simulink model "task_4_sim"  (R2023a)
settings: Solver=VariableStepAuto  StartTime=0.0  StopTime=10.0  RelTol=1e-3
undefined symbols (not defined in the file): A, B, Cz, Dz, G, K1, K2, w0
settings Model: Creator=user  LastModifiedBy=user

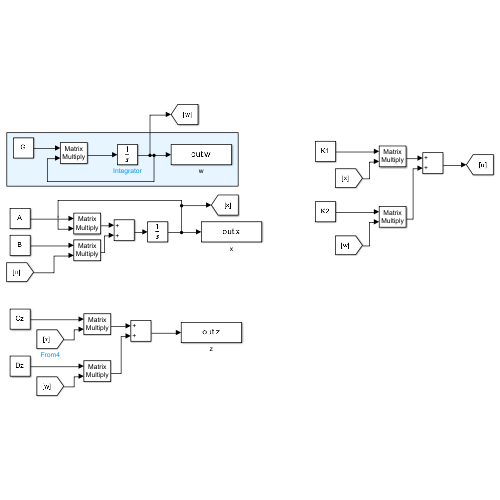
[thumbnail: Simulink's stored preview of the top-level diagram]
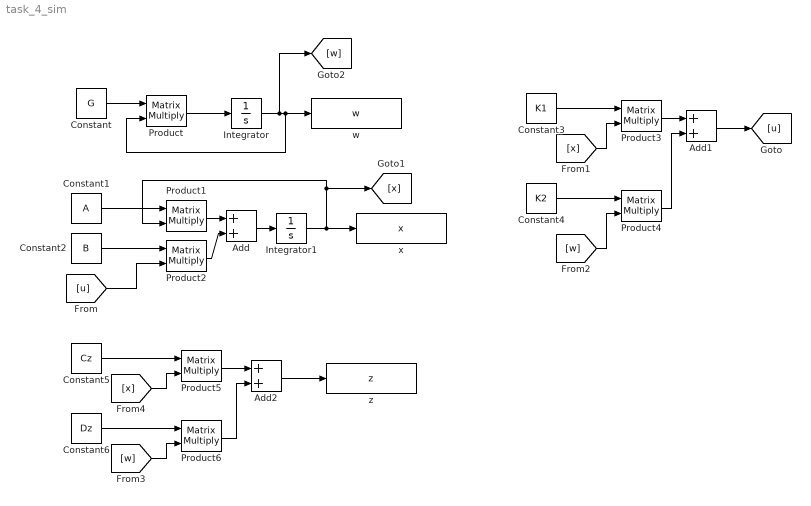
== system task_4_sim ==
  Add : Sum
  Add1 : Sum
  Add2 : Sum
  Constant : Constant  Value=G  VectorParams1D=off
  Constant1 : Constant  Value=A  VectorParams1D=off
  Constant2 : Constant  Value=B
  Constant3 : Constant  Value=K1  VectorParams1D=off
  Constant4 : Constant  Value=K2
  Constant5 : Constant  Value=Cz  VectorParams1D=off
  Constant6 : Constant  Value=Dz  VectorParams1D=off
  Integrator : Integrator  InitialCondition=w0
  Integrator1 : Integrator
  Product{,1..6} (7 alike) : Product  Multiplication=Matrix(*)
  w : ToWorkspace  VariableName=w  SaveFormat=Timeseries  SampleTime=-1
  x : ToWorkspace  VariableName=x  SaveFormat=Timeseries  SampleTime=-1
  z : ToWorkspace  VariableName=z  SaveFormat=Timeseries  SampleTime=-1
  wires:
  Integrator/1 -> [w], Product/2, w/1
  Product/1 -> Integrator/1
  Constant/1 -> Product/1
  Integrator1/1 -> x/1, [x], Product1/2
  Constant1/1 -> Product1/1
  Constant2/1 -> Product2/1
  Product1/1 -> Add/1
  Add/1 -> Integrator1/1
  Product2/1 -> Add/2
  [u] -> Product2/2
  Add1/1 -> [u]
  Constant4/1 -> Product4/1
  Constant3/1 -> Product3/1
  [x] -> Product3/2
  Product3/1 -> Add1/1
  [w] -> Product4/2
  Product4/1 -> Add1/2
  Constant5/1 -> Product5/1
  [x] -> Product5/2
  Constant6/1 -> Product6/1
  [w] -> Product6/2
  Product5/1 -> Add2/1
  Product6/1 -> Add2/2
  Add2/1 -> z/1
